simulink model "sederhana"  (R2023b)
settings: Solver=VariableStepAuto  StartTime=0.0  StopTime=10.0  RelTol=1e-3
libraries: simulink x2
settings Model: Creator=NITRO  LastModifiedBy=NITRO

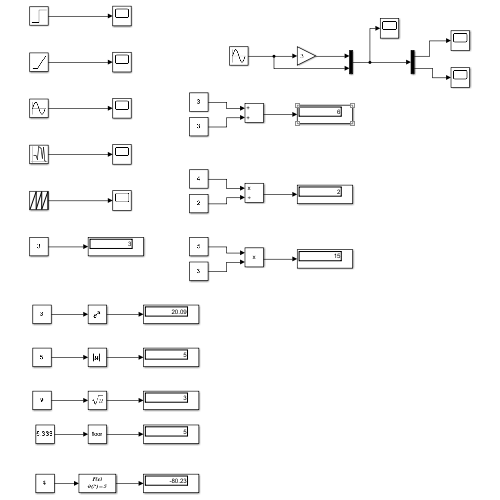
[thumbnail: Simulink's stored preview of the top-level diagram]
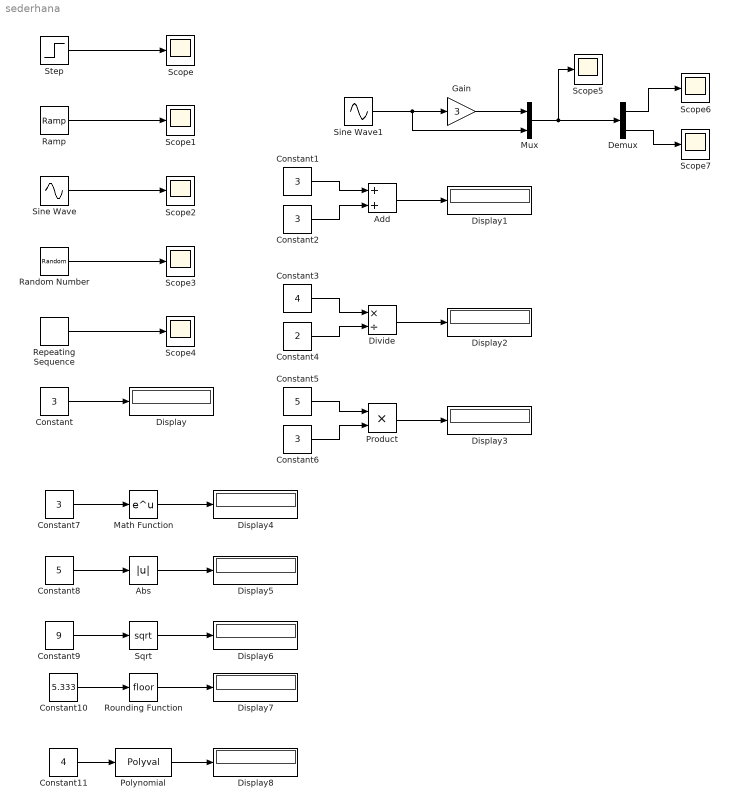
== system sederhana ==
  Abs : Abs  SaturateOnIntegerOverflow=off
  Add : Sum
  Constant{,1..2,6..7} (5 alike) : Constant  Value=3
  Constant10 : Constant  Value=5.333
  Constant11 : Constant  Value=4
  Constant3 : Constant  Value=4
  Constant4 : Constant  Value=2
  Constant5 : Constant  Value=5
  Constant8 : Constant  Value=5
  Constant9 : Constant  Value=9
  Demux : Demux  Outputs=2
  Display{,1..8} (9 alike) : Display
  Divide : Product  Inputs=*/
  Gain : Gain  Gain=3
  Math Function : Math
  Mux : Mux  Inputs=2
  Polynomial : Polyval  Coefs=[ +2.081618890e-019, -1.441693666e-014, +4.719686976e-010, -8.536869453e-006, +1.621573104e-001, -8.087801117e+001 ]
  Product : Product
  Ramp : simulink/Sources/Ramp  slope=3  start=0  InitialOutput=0
  Random Number : RandomNumber  SampleTime=1
  Repeating Sequence : simulink/Sources/Repeating Sequence  rep_seq_t=[0 1]  rep_seq_y=[0 1]
  Rounding Function : Rounding
  Scope{,1..7} (8 alike) : Scope
  Sine Wave : Sin  Amplitude=3  Frequency=2  SampleTime=0
  Sine Wave1 : Sin  SampleTime=0
  Sqrt : Sqrt
  Step : Step  Time=3  After=5  SampleTime=0
  wires:
  Step/1 -> Scope/1
  Ramp/1 -> Scope1/1
  Sine Wave/1 -> Scope2/1
  Random Number/1 -> Scope3/1
  Repeating Sequence/1 -> Scope4/1
  Constant/1 -> Display/1
  Gain/1 -> Mux/1
  Sine Wave1/1 -> Mux/2, Gain/1
  Mux/1 -> Scope5/1, Demux/1
  Demux/1 -> Scope6/1
  Demux/2 -> Scope7/1
  Constant3/1 -> Divide/1
  Constant4/1 -> Divide/2
  Constant1/1 -> Add/1
  Constant2/1 -> Add/2
  Add/1 -> Display1/1
  Divide/1 -> Display2/1
  Constant5/1 -> Product/1
  Constant6/1 -> Product/2
  Product/1 -> Display3/1
  Constant11/1 -> Polynomial/1
  Constant10/1 -> Rounding Function/1
  Constant9/1 -> Sqrt/1
  Constant8/1 -> Abs/1
  Constant7/1 -> Math Function/1
  Math Function/1 -> Display4/1
  Abs/1 -> Display5/1
  Sqrt/1 -> Display6/1
  Rounding Function/1 -> Display7/1
  Polynomial/1 -> Display8/1
